simulink model "ex2_12"  (R2019a)
settings: Solver=VariableStepAuto  StartTime=0.0  StopTime=5  RelTol=1e-3
settings Model: Creator=Lenovo  LastModifiedBy=Lenovo

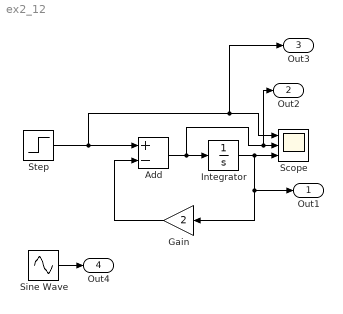
== system ex2_12 ==
  Add : Sum  Inputs=+-
  Gain : Gain  Gain=2
  Integrator : Integrator
  Scope : Scope  NumInputPorts=3
  Sine Wave : Sin  SampleTime=0
  Step : Step  SampleTime=0
  Out1 : Outport  SignalName=y3
  Out2 : Outport  Port=2  SignalName=y2
  Out3 : Outport  Port=3  SignalName=y1
  Out4 : Outport  Port=4
  wires:
  Step/1 -> Out3/1, Scope/1, Add/1
  Gain/1 -> Add/2
  Add/1 -> Out2/1, Scope/2, Integrator/1
  Integrator/1 -> Out1/1, Gain/1, Scope/3
  Sine Wave/1 -> Out4/1
